simulink model "simple"  (R2018a)
settings: Solver=VariableStepAuto  StartTime=0.0  StopTime=10.0  RelTol=1e-3
settings Model: Creator=ishaf  LastModifiedBy=ishaf

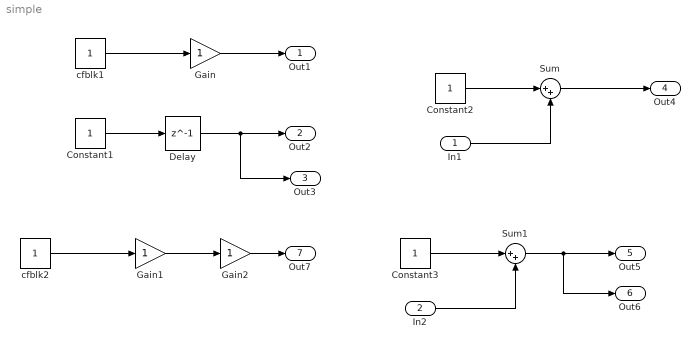
== system simple ==
  In1 : Inport
  In2 : Inport  Port=2
  Constant1 : Constant
  Constant2 : Constant
  Constant3 : Constant
  Delay : Delay  DelayLength=1  InitialCondition=0
  Gain : Gain
  Gain1 : Gain
  Gain2 : Gain
  Sum : Sum  Inputs=|++
  Sum1 : Sum  Inputs=|++
  cfblk1 : Constant
  cfblk2 : Constant
  Out1 : Outport
  Out2 : Outport  Port=2
  Out3 : Outport  Port=3
  Out4 : Outport  Port=4
  Out5 : Outport  Port=5
  Out6 : Outport  Port=6
  Out7 : Outport  Port=7
  wires:
  cfblk1/1 -> Gain/1
  Gain/1 -> Out1/1
  Constant1/1 -> Delay/1
  Delay/1 -> Out3/1, Out2/1
  Constant2/1 -> Sum/1
  In1/1 -> Sum/2
  Sum/1 -> Out4/1
  Sum1/1 -> Out6/1, Out5/1
  In2/1 -> Sum1/2
  Constant3/1 -> Sum1/1
  cfblk2/1 -> Gain1/1
  Gain1/1 -> Gain2/1
  Gain2/1 -> Out7/1
